simulink model "water_control"  (R2018b)
settings: Solver=VariableStepAuto  StartTime=0.0  StopTime=500  RelTol=1e-3
values from neighbouring files (symbols this model uses):
  level0 = 0    [waterBreach.m]
  level_inc = v_flow / (15 * 15)    (= 1)    [waterBreach.m]
settings Model: Creator=miokey  LastModifiedBy=miokey

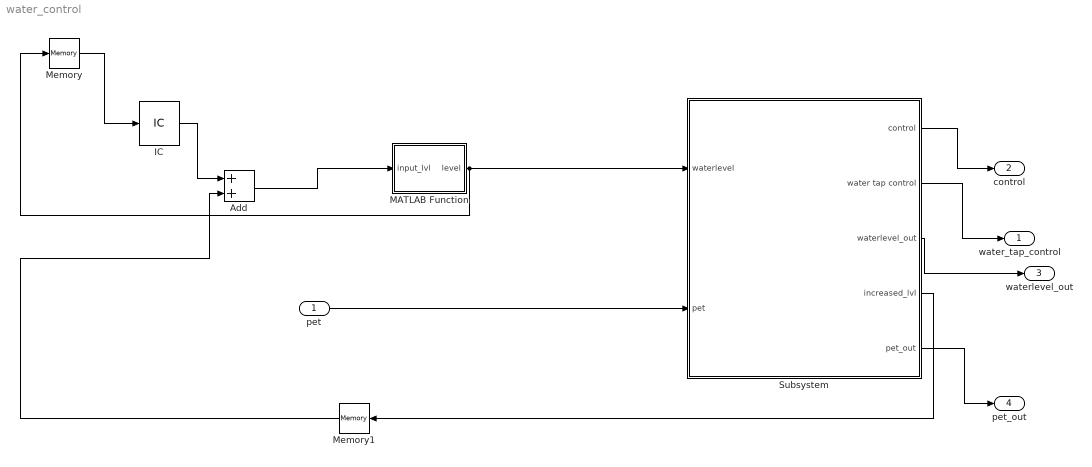
== system water_control ==
  "pet " : Inport
  Add : Sum
  IC : InitialCondition  Value=level0
  MATLAB Function : MATLAB Function  TreatAsAtomicUnit=on
  Memory : Memory
  Memory1 : Memory
  Subsystem : Subsystem
  water_tap_control : Outport
  control : Outport  Port=2
  waterlevel_out : Outport  Port=3
  "pet_out " : Outport  Port=4
  wires:
  "pet "/1 -> Subsystem/2("pet ")
  Add/1 -> MATLAB Function/1(input_lvl)
  Subsystem/2("water tap control ") -> water_tap_control/1
  Subsystem/1(control) -> control/1
  Subsystem/3(waterlevel_out) -> waterlevel_out/1
  IC/1 -> Add/1
  Memory/1 -> IC/1
  Memory1/1 -> Add/2
  Subsystem/4("increased_lvl ") -> Memory1/1
  MATLAB Function/1(level) -> Memory/1, Subsystem/1(waterlevel)
  Subsystem/5("pet_out ") -> "pet_out "/1

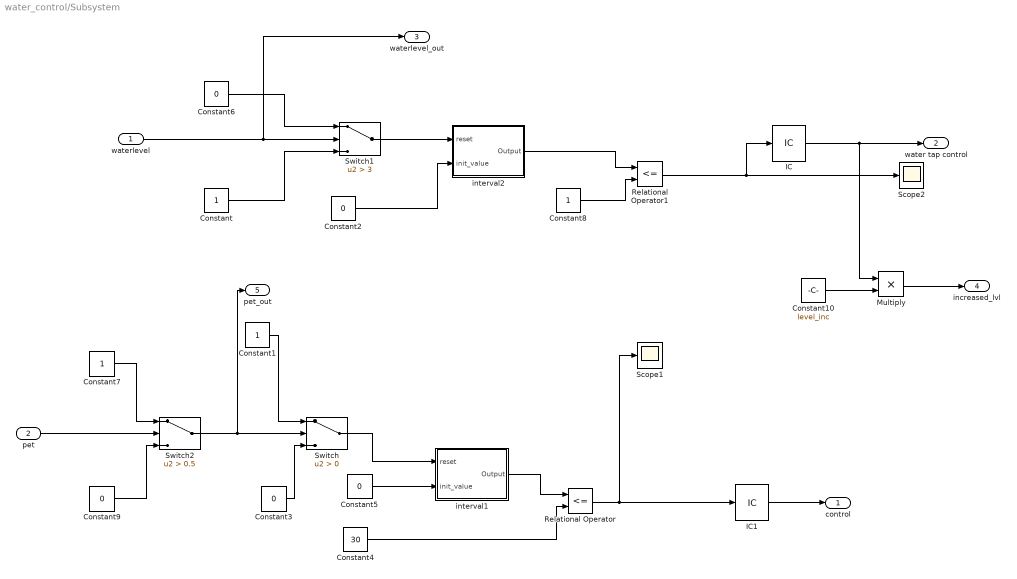
== system water_control/Subsystem ==
  waterlevel : Inport
  "pet " : Inport  Port=2
  Constant{,1,7..8} (4 alike) : Constant
  Constant10 : Constant  Value=level_inc
  Constant{2..3,5..6,9} (5 alike) : Constant  Value=0
  Constant4 : Constant  Value=30
  IC : InitialCondition  Value=0
  IC1 : InitialCondition  Value=0
  Multiply : Product
  Relational Operator : RelationalOperator  Operator=<=  OutDataTypeStr=boolean  RndMeth=Simplest
  Relational Operator1 : RelationalOperator  Operator=<=  OutDataTypeStr=boolean  RndMeth=Simplest
  Scope1 : Scope
  Scope2 : Scope
  Switch : Switch  Criteria=u2 > Threshold
  Switch1 : Switch  Criteria=u2 > Threshold  Threshold=3
  Switch2 : Switch  Criteria=u2 > Threshold  Threshold=0.5
  interval1 : Subsystem
  interval2 : Subsystem
  control : Outport
  "water tap control " : Outport  Port=2
  waterlevel_out : Outport  Port=3
  "increased_lvl " : Outport  Port=4
  "pet_out " : Outport  Port=5
  wires:
  Constant6/1 -> Switch1/1
  Constant/1 -> Switch1/3
  Constant5/1 -> interval1/2(init_value)
  interval1/1(Output) -> Relational Operator/1
  Relational Operator/1 -> IC1/1, Scope1/1
  Constant4/1 -> Relational Operator/2
  Constant1/1 -> Switch/1
  Switch/1 -> interval1/1(reset)
  Constant3/1 -> Switch/3
  waterlevel/1 -> waterlevel_out/1, Switch1/2
  Relational Operator1/1 -> IC/1, Scope2/1
  Constant8/1 -> Relational Operator1/2
  Switch1/1 -> interval2/1(reset)
  interval2/1(Output) -> Relational Operator1/1
  Constant2/1 -> interval2/2(init_value)
  "pet "/1 -> Switch2/2
  Constant7/1 -> Switch2/1
  Constant9/1 -> Switch2/3
  Switch2/1 -> "pet_out "/1, Switch/2
  Constant10/1 -> Multiply/2
  Multiply/1 -> "increased_lvl "/1
  IC/1 -> Multiply/1, "water tap control "/1
  IC1/1 -> control/1

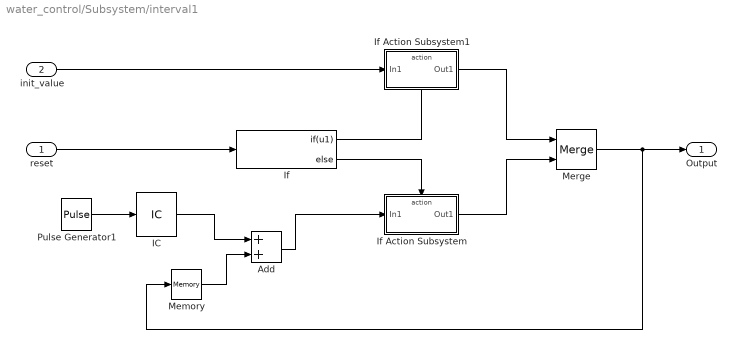
== system water_control/Subsystem/interval1 ==
  reset : Inport
  init_value : Inport  Port=2
  Add : Sum
  IC : InitialCondition  Value=30
  If : If  IfExpression=u1
  If Action Subsystem : Subsystem  TreatAsAtomicUnit=on
  If Action Subsystem1 : Subsystem  TreatAsAtomicUnit=on
  Memory : Memory
  Merge : Merge
  Pulse Generator1 : DiscretePulseGenerator  PulseType=Time based  Period=1  PulseWidth=5  PhaseDelay=1
  Output : Outport
  wires:
  If/2 -> If Action Subsystem/Action
  If Action Subsystem1/1(Out1) -> Merge/1
  Merge/1 -> Output/1, Memory/1
  init_value/1 -> If Action Subsystem1/1(In1)
  Add/1 -> If Action Subsystem/1(In1)
  Memory/1 -> Add/2
  If/1 -> If Action Subsystem1/Action
  If Action Subsystem/1(Out1) -> Merge/2
  reset/1 -> If/1
  Pulse Generator1/1 -> IC/1
  IC/1 -> Add/1

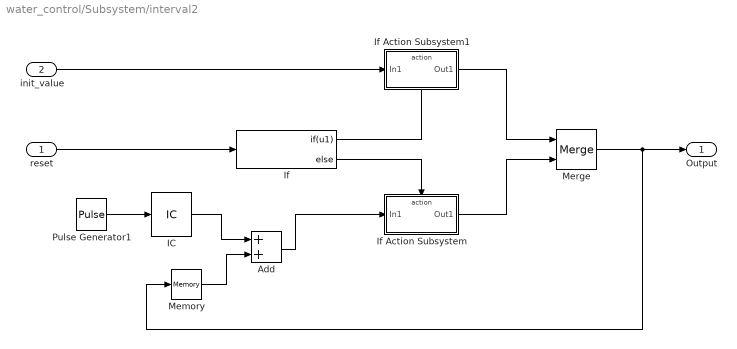
== system water_control/Subsystem/interval2 ==
  reset : Inport
  init_value : Inport  Port=2
  Add : Sum
  IC : InitialCondition  Value=3
  If : If  IfExpression=u1
  If Action Subsystem : Subsystem  TreatAsAtomicUnit=on
  If Action Subsystem1 : Subsystem  TreatAsAtomicUnit=on
  Memory : Memory
  Merge : Merge
  Pulse Generator1 : DiscretePulseGenerator  PulseType=Time based  Period=1  PulseWidth=5  PhaseDelay=1
  Output : Outport
  wires:
  If/2 -> If Action Subsystem/Action
  If Action Subsystem1/1(Out1) -> Merge/1
  Merge/1 -> Output/1, Memory/1
  init_value/1 -> If Action Subsystem1/1(In1)
  Add/1 -> If Action Subsystem/1(In1)
  Memory/1 -> Add/2
  If/1 -> If Action Subsystem1/Action
  If Action Subsystem/1(Out1) -> Merge/2
  reset/1 -> If/1
  Pulse Generator1/1 -> IC/1
  IC/1 -> Add/1

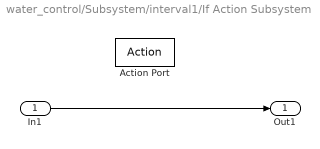
== system water_control/Subsystem/interval1/If Action Subsystem ==
  In1 : Inport
  Action Port : ActionPort  ActionType=else
  Out1 : Outport
  wires:
  In1/1 -> Out1/1

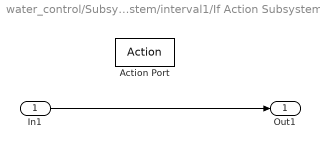
== system water_control/Subsystem/interval1/If Action Subsystem1 ==
  In1 : Inport
  Action Port : ActionPort  ActionType=then
  Out1 : Outport
  wires:
  In1/1 -> Out1/1

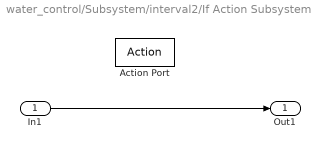
== system water_control/Subsystem/interval2/If Action Subsystem ==
  In1 : Inport
  Action Port : ActionPort
  Out1 : Outport
  wires:
  In1/1 -> Out1/1

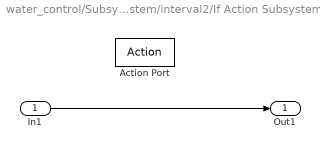
== system water_control/Subsystem/interval2/If Action Subsystem1 ==
  In1 : Inport
  Action Port : ActionPort
  Out1 : Outport
  wires:
  In1/1 -> Out1/1

== matlab function water_control/MATLAB Function ==
  data: input_lvl input; level output
function level = fcn(input_lvl)

level = input_lvl - abs(rand() - 0.5);
